simulink model "mvdc_mpc"  (R2018b)
settings: configuration reference "Active" (kept outside this file)
undefined symbols (not defined in the file): A_VehicleReference_m2, acc_control_learning, ax_lim_mps2, ay_lim_mps2, DiscIntNeverNeededParam, drag_coefficient, l_front_m, l_rear_m, LatAcc_cov_debug, LatAcc_FFweights, LatAcc_mean_debug, LongAcc_FFweights, P_VDC_axFFModelLearningEnable, P_VDC_axFFModelLearningRate, P_VDC_axFFModelLearningReg, P_VDC_ayFFModelLearningEnable, P_VDC_ayFFModelLearningRate, P_VDC_ayFFModelLearningReg, P_VDC_Dist_ax_perc, P_VDC_Dist_ay_perc, P_VDC_EnableNumLatErrorDer_b, P_VDC_EnableTubeMPC, P_VDC_EnableUncertaintyLearning, P_VDC_EnableYawRateAccRepl, P_VDC_LatAcc_BetaGain, P_VDC_LatAcc_EnableForesightFF, P_VDC_LatAcc_FF_Ts, P_VDC_LatAcc_Steering_Ts, P_VDC_LatAcc_UndersteerComp_Ts, P_VDC_LatAcc_VehicleDynamics_Ts, P_VDC_LatAccKi, P_VDC_LatAccKi_Lim_perc, P_VDC_LatAccKp_ay, P_VDC_LatAccKp_Delta, P_VDC_LatErrorDer_Ts_s, P_VDC_LongAcc_EnableForesightFF, P_VDC_LongAcc_FB_Ts, P_VDC_LongAcc_FF_Ts, P_VDC_LongAcc_LimFb_N, P_VDC_LongAccKp, P_VDC_MaxTightening, P_VDC_MinVelSlipCalc_mps, P_VDC_PositiveAxLimScale, P_VDC_StabilizerRearSideSlip_rad, P_VDC_SteeringOvalComp_rad, P_VDC_SteeringSteadyStateUndersteerComp_rad, P_VDC_UncertaintyLearningGain, P_VDC_UncertaintyLearningSamples, P_VDC_UncertaintyTarget_perc, P_VDC_VirtualController, Pos, roh_air, sys, tS, tSSlow, TUMHealthStatus, v_mps, vehiclemass_kg
libraries: simulink x31
(part 2 of 2)

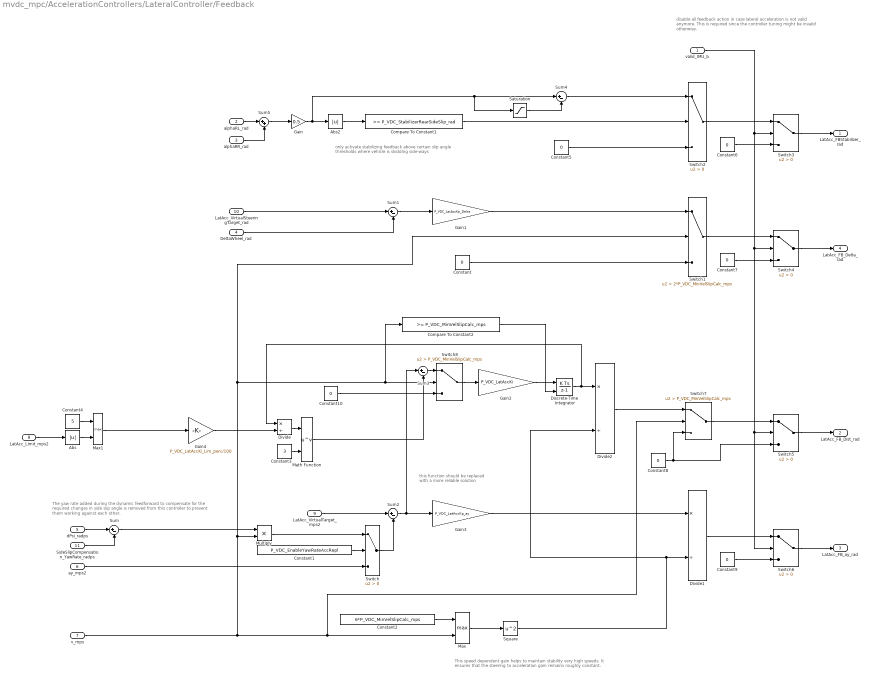
== system mvdc_mpc/AccelerationControllers/LateralController/Feedback ==
  note: disable all feedback action in case
      | lateral acceleration is not valid anymore.
      |
      | This is required since the controller tuning might be invalid otherwise.
  note: only activate stabilizing feedback above certain slip angle
      | thresholds where vehicle is skidding side-ways
  note: this function should be replaced
      | with a more reliable solution
  note: The yaw rate added during the dynamic feedforward to compensate
      | for the required changes in side slip angle is removed from this controller
      | to prevent them working against each other.
  note: This speed dependent gain helps to maintain stability very high speeds.
      | It ensures that the steering to acceleration gain remains roughly constant.
  valid_IMU_b : Inport
  alphaRL_rad : Inport  Port=2
  alphaRR_rad : Inport  Port=3
  DeltaWheel_rad : Inport  Port=4
  dPsi_radps : Inport  Port=5
  ay_mps2 : Inport  Port=6
  v_mps : Inport  Port=7
  LatAcc_Limit_mps2 : Inport  Port=8
  LatAcc_VirtualTarget_mps2 : Inport  Port=9
  LatAcc_VirtualSteeringTarget_rad : Inport  Port=10
  SideSlipCompensation_YawRate_radps : Inport  Port=11
  Abs : Abs
  Abs2 : Abs
  Compare To Constant1 : simulink/Logic and Bit Operations/Compare To Constant  relop=>=  const=P_VDC_StabilizerRearSideSlip_rad  OutDataTypeStr=boolean
  Compare To Constant2 : simulink/Logic and Bit Operations/Compare To Constant  relop=>=  const=P_VDC_MinVelSlipCalc_mps  OutDataTypeStr=boolean
  Constant{,5..10} (7 alike) : Constant  Value=0
  Constant1 : Constant  Value=P_VDC_EnableYawRateAccRepl
  Constant2 : Constant  Value=6*P_VDC_MinVelSlipCalc_mps
  Constant3 : Constant  Value=3
  Constant4 : Constant  Value=5
  Discrete-Time Integrator : DiscreteIntegrator  ExternalReset=falling  SampleTime=-1  ICPrevOutput=DiscIntNeverNeededParam  ICPrevScaledInput=DiscIntNeverNeededParam
  Divide : Product  Inputs=*/
  Divide1 : Product  Inputs=*/
  Divide2 : Product  Inputs=*/
  Gain : Gain  Gain=0.5
  Gain1 : Gain  Gain=P_VDC_LatAccKp_Delta
  Gain2 : Gain  Gain=P_VDC_LatAccKi
  Gain3 : Gain  Gain=P_VDC_LatAccKp_ay
  Gain4 : Gain  Gain=P_VDC_LatAccKi_Lim_perc/100
  Math Function : Math  Operator=pow  SaturateOnIntegerOverflow=on
  Max : MinMax  Function=max  Inputs=2
  Max1 : MinMax  Function=max  Inputs=2
  Multiply : Product
  Saturation : Saturate  UpperLimit=P_VDC_StabilizerRearSideSlip_rad  LowerLimit=-P_VDC_StabilizerRearSideSlip_rad
  Square : Math  Operator=square  SaturateOnIntegerOverflow=on
  Sum{,1..4} (5 alike) : Sum  Inputs=|+-
  Sum5 : Sum  Inputs=|++
  Switch{,2..6} (6 alike) : Switch  Criteria=u2 > Threshold
  Switch1 : Switch  Criteria=u2 > Threshold  Threshold=2*P_VDC_MinVelSlipCalc_mps
  Switch7 : Switch  Criteria=u2 > Threshold  Threshold=P_VDC_MinVelSlipCalc_mps
  Switch8 : Switch  Criteria=u2 > Threshold  Threshold=P_VDC_MinVelSlipCalc_mps
  LatAcc_FBStabilizer_rad : Outport
  LatAcc_FB_Dist_rad : Outport  Port=2
  LatAcc_FB_ay_rad : Outport  Port=3
  LatAcc_FB_Delta_rad : Outport  Port=4
  wires:
  Gain3/1 -> Divide1/1
  Constant2/1 -> Max/1
  Square/1 -> Divide2/2, Divide1/2
  v_mps/1 -> Compare To Constant2/1, Switch8/2, Switch1/2, Multiply/2, Switch7/2, Max/2
  Max/1 -> Square/1
  Multiply/1 -> Switch/1
  ay_mps2/1 -> Switch/3
  Constant1/1 -> Switch/2
  dPsi_radps/1 -> Sum/1
  SideSlipCompensation_YawRate_radps/1 -> Sum/2
  Sum/1 -> Multiply/1
  Switch/1 -> Sum2/2
  LatAcc_VirtualSteeringTarget_rad/1 -> Sum1/1
  DeltaWheel_rad/1 -> Sum1/2
  Sum1/1 -> Gain1/1
  Gain1/1 -> Switch1/1
  Constant/1 -> Switch1/3
  Discrete-Time Integrator/1 -> Divide/1, Divide2/1
  Sum2/1 -> Sum3/1, Gain3/1
  Gain4/1 -> Divide/2
  Divide/1 -> Math Function/1
  Constant3/1 -> Math Function/2
  Max1/1 -> Gain4/1
  Abs/1 -> Max1/2
  LatAcc_VirtualTarget_mps2/1 -> Sum2/1
  Constant4/1 -> Max1/1
  Gain2/1 -> Discrete-Time Integrator/1
  Math Function/1 -> Sum3/2
  Constant5/1 -> Switch2/3
  Abs2/1 -> Compare To Constant1/1
  Sum4/1 -> Switch2/1
  Gain/1 -> Saturation/1, Sum4/1, Abs2/1
  Saturation/1 -> Sum4/2
  Compare To Constant1/1 -> Switch2/2
  LatAcc_Limit_mps2/1 -> Abs/1
  alphaRL_rad/1 -> Sum5/1
  alphaRR_rad/1 -> Sum5/2
  Sum5/1 -> Gain/1
  Switch2/1 -> Switch3/1
  Switch3/1 -> LatAcc_FBStabilizer_rad/1
  Switch1/1 -> Switch4/1
  Switch4/1 -> LatAcc_FB_Delta_rad/1
  Switch5/1 -> LatAcc_FB_Dist_rad/1
  Divide1/1 -> Switch6/1
  Switch6/1 -> LatAcc_FB_ay_rad/1
  valid_IMU_b/1 -> Switch6/2, Switch5/2, Switch4/2, Switch3/2
  Constant6/1 -> Switch3/3
  Constant7/1 -> Switch4/3
  Constant8/1 -> Switch5/3, Switch7/3
  Constant9/1 -> Switch6/3
  Switch7/1 -> Switch5/1
  Divide2/1 -> Switch7/1
  Switch8/1 -> Gain2/1
  Sum3/1 -> Switch8/1
  Constant10/1 -> Switch8/3
  Compare To Constant2/1 -> Discrete-Time Integrator/2

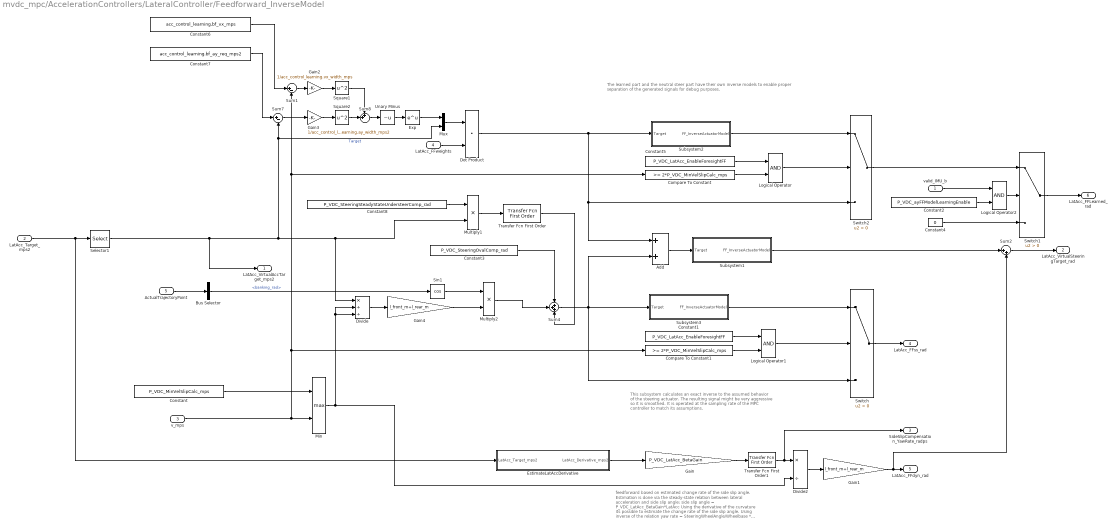
== system mvdc_mpc/AccelerationControllers/LateralController/Feedforward_InverseModel ==
  note: The learned part and the neutral steer part have their own
      | inverse models to enable proper separation of the generated signals for debug purposes.
  note: This subsystem calculates an exact inverse
      | to the assumed behavior of the steering actuator.
      | The resulting signal might be very aggressive so it is smoothed.
      | It is operated at the sampling rate of the MPC controller to match
      | its assumptions.
  note: feedforward based on estimated change rate
      | of the side slip angle. Estimation is done via the steady-state
      | relation between lateral acceleration and side slip angle:
      |
      | side slip angle = P_VDC_LatAcc_BetaGain*LatAcc
      |
      | Using the derivative of the curvature its possible to estimate the
      | change rate of the side slip angle. Using inverse of the relation
      |
      | yaw rate = SteeringWheelAngle/Wheelbase * Velocity
      |
      | we can calculate a compensation yaw rate and the corresponding
      | steering wheel angle.
  valid_IMU_b : Inport
  LatAcc_Target_mps2 : Inport  Port=2
  v_mps : Inport  Port=3
  LatAcc_FFweights : Inport  Port=4
  ActualTrajectoryPoint : Inport  Port=5
  Add : Sum
  Bus Selector : BusSelector  OutputSignals=banking_rad
  Compare To Constant : simulink/Logic and Bit Operations/Compare To Constant  relop=>=  const=2*P_VDC_MinVelSlipCalc_mps  OutDataTypeStr=boolean
  Compare To Constant1 : simulink/Logic and Bit Operations/Compare To Constant  relop=>=  const=2*P_VDC_MinVelSlipCalc_mps  OutDataTypeStr=boolean
  Constant : Constant  Value=P_VDC_MinVelSlipCalc_mps
  Constant1 : Constant  Value=P_VDC_LatAcc_EnableForesightFF
  Constant2 : Constant  Value=P_VDC_ayFFModelLearningEnable
  Constant3 : Constant  Value=P_VDC_SteeringOvalComp_rad
  Constant4 : Constant  Value=0
  Constant5 : Constant  Value=P_VDC_LatAcc_EnableForesightFF
  Constant6 : Constant  Value=acc_control_learning.bf_vx_mps
  Constant7 : Constant  Value=acc_control_learning.bf_ay_req_mps2
  Constant8 : Constant  Value=P_VDC_SteeringSteadyStateUndersteerComp_rad
  Divide : Product  Inputs=*//
  Divide2 : Product  Inputs=*/
  Dot Product : DotProduct  InputSameDT=on  OutDataTypeStr=Inherit: Inherit via internal rule
  EstimateLatAccDerivative : Subsystem
  Exp : Math  SaturateOnIntegerOverflow=on
  Gain : Gain  Gain=P_VDC_LatAcc_BetaGain
  Gain1 : Gain  Gain=l_front_m+l_rear_m
  Gain2 : Gain  Gain=1/acc_control_learning.vx_width_mps
  Gain3 : Gain  Gain=1/acc_control_learning.ay_width_mps2
  Gain4 : Gain  Gain=l_front_m+l_rear_m
  Logical Operator : Logic  AllPortsSameDT=off  OutDataTypeStr=boolean
  Logical Operator1 : Logic  AllPortsSameDT=off  OutDataTypeStr=boolean
  Logical Operator2 : Logic  AllPortsSameDT=off  OutDataTypeStr=boolean
  Min : MinMax  Function=max  Inputs=2
  Multiply1 : Product
  Multiply2 : Product
  Mux : Mux  Inputs=2
  Selector1 : Selector  InputPortWidth=sys.N_hor+1  IndexOptions=Index vector (dialog)  Indices=1  OutputSizes=1
  Sin1 : Trigonometry  Operator=cos
  Square1 : Math  Operator=square  SaturateOnIntegerOverflow=on
  Square2 : Math  Operator=square  SaturateOnIntegerOverflow=on
  Subsystem1 : Subsystem  SystemSampleTime=tSSlow
  Subsystem2 : Subsystem  SystemSampleTime=tSSlow
  Subsystem3 : Subsystem  SystemSampleTime=tSSlow
  Sum1 : Sum  Inputs=|+-
  Sum2 : Sum  Inputs=|++
  Sum4 : Sum  Inputs=+++
  Sum7 : Sum  Inputs=|+-
  Sum8 : Sum  Inputs=++|
  Switch : Switch  Criteria=u2 > Threshold
  Switch1 : Switch  Criteria=u2 > Threshold
  Switch2 : Switch  Criteria=u2 > Threshold
  Transfer Fcn First Order : simulink/Discrete/Transfer Fcn First Order  PoleZ=exp(-tS/P_VDC_LatAcc_UndersteerComp_Ts)  ICPrevOutput=0.0  DoSatur=off
      settings: SourceProductName=Simulink
  Transfer Fcn First Order1 : simulink/Discrete/Transfer Fcn First Order  PoleZ=exp(-tS/P_VDC_LatAcc_FF_Ts)  ICPrevOutput=0.0  DoSatur=off
      settings: SourceProductName=Simulink
  Unary Minus : UnaryMinus
  LatAcc_VirtualAccTarget_mps2 : Outport
  LatAcc_VirtualSteeringTarget_rad : Outport  Port=2
  SideSlipCompensation_YawRate_radps : Outport  Port=3
  LatAcc_FFss_rad : Outport  Port=4
  LatAcc_FFdyn_rad : Outport  Port=5
  LatAcc_FFLearned_rad : Outport  Port=6
  wires:
  Constant/1 -> Min/1
  LatAcc_Target_mps2/1 -> Selector1/1, EstimateLatAccDerivative/1(LatAcc_Target_mps2)
  Logical Operator1/1 -> Switch/2
  EstimateLatAccDerivative/1(LatAcc_Derivative_mps2) -> Gain/1
  Min/1 -> Divide2/2, Divide/3, Divide/2
  Transfer Fcn First Order1/1 -> SideSlipCompensation_YawRate_radps/1, Divide2/1
  Divide/1 -> Gain4/1
  Divide2/1 -> Gain1/1
  Gain/1 -> Transfer Fcn First Order1/1
  Gain1/1 -> Sum2/2, LatAcc_FFdyn_rad/1
  Switch1/1 -> LatAcc_FFLearned_rad/1
  Constant4/1 -> Switch1/3
  Switch/1 -> LatAcc_FFss_rad/1
  Subsystem2/1(FF_InverseActuatorModel) -> Switch2/1
  Dot Product/1 -> Subsystem2/1(Target), Add/1, Switch2/3
  Switch2/1 -> Switch1/1
  Square1/1 -> Sum8/1
  Sum8/1 -> Unary Minus/1
  Gain3/1 -> Square2/1
  Gain2/1 -> Square1/1
  Square2/1 -> Sum8/2
  LatAcc_FFweights/1 -> Dot Product/2
  Sum1/1 -> Gain2/1
  Sum7/1 -> Gain3/1
  Unary Minus/1 -> Exp/1
  Exp/1 -> Mux/1
  Constant6/1 -> Sum1/1
  Constant7/1 -> Sum7/1
  v_mps/1 -> Min/2, Compare To Constant1/1, Compare To Constant/1, Sum1/2
  Mux/1 -> Dot Product/1
  Sum4/1 -> Subsystem3/1(Target), Add/2, Switch/3
  Subsystem3/1(FF_InverseActuatorModel) -> Switch/1
  Subsystem1/1(FF_InverseActuatorModel) -> Sum2/1
  Add/1 -> Subsystem1/1(Target)
  Sum2/1 -> LatAcc_VirtualSteeringTarget_rad/1
  Constant5/1 -> Logical Operator/1
  Logical Operator/1 -> Switch2/2
  Compare To Constant/1 -> Logical Operator/2
  Constant1/1 -> Logical Operator1/1
  Compare To Constant1/1 -> Logical Operator1/2
  Logical Operator2/1 -> Switch1/2
  Constant2/1 -> Logical Operator2/2
  valid_IMU_b/1 -> Logical Operator2/1
  Constant3/1 -> Sum4/1
  Constant8/1 -> Multiply1/1
  Multiply1/1 -> Transfer Fcn First Order/1
  Transfer Fcn First Order/1 -> Sum4/3
  ActualTrajectoryPoint/1 -> Bus Selector/1
  Selector1/1 -> LatAcc_VirtualAccTarget_mps2/1, Sum7/2, Mux/2, Multiply1/2, Divide/1  "Target"
  Gain4/1 -> Multiply2/2
  Multiply2/1 -> Sum4/2
  Sin1/1 -> Multiply2/1
  Bus Selector/1 -> Sin1/1  "<banking_rad>"

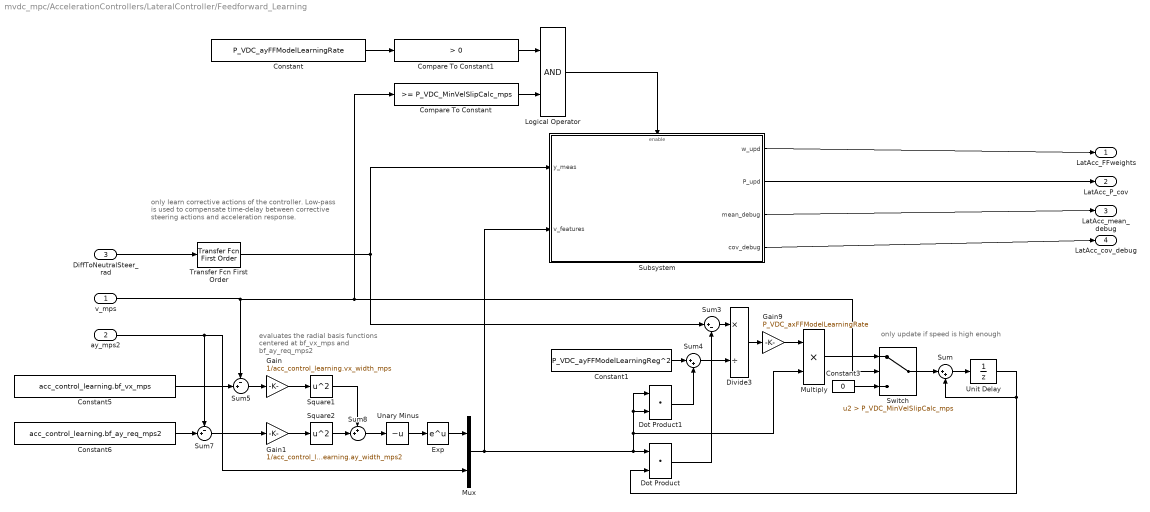
== system mvdc_mpc/AccelerationControllers/LateralController/Feedforward_Learning ==
  note: evaluates the radial
      | basis functions centered at
      | bf_vx_mps and bf_ay_req_mps2
  note: only learn corrective actions of the controller.
      | Low-pass is used to compensate time-delay
      | between corrective steering actions and acceleration
      | response.
  note: only update if speed is high enough
  v_mps : Inport
  ay_mps2 : Inport  Port=2
  DiffToNeutralSteer_rad : Inport  Port=3
  Compare To Constant : simulink/Logic and Bit Operations/Compare To Constant  relop=>=  const=P_VDC_MinVelSlipCalc_mps  OutDataTypeStr=boolean
  Compare To Constant1 : simulink/Logic and Bit Operations/Compare To Constant  relop=>  const=0  OutDataTypeStr=boolean
  Constant : Constant  Value=P_VDC_ayFFModelLearningRate
  Constant1 : Constant  Value=P_VDC_ayFFModelLearningReg^2
  Constant3 : Constant  Value=0
  Constant5 : Constant  Value=acc_control_learning.bf_vx_mps
  Constant6 : Constant  Value=acc_control_learning.bf_ay_req_mps2
  Divide3 : Product  Inputs=*/
  Dot Product : DotProduct  InputSameDT=on  OutDataTypeStr=Inherit: Inherit via internal rule
  Dot Product1 : DotProduct  InputSameDT=on  OutDataTypeStr=Inherit: Inherit via internal rule
  Exp : Math  SaturateOnIntegerOverflow=on
  Gain : Gain  Gain=1/acc_control_learning.vx_width_mps
  Gain1 : Gain  Gain=1/acc_control_learning.ay_width_mps2
  Gain9 : Gain  Gain=P_VDC_axFFModelLearningRate
  Logical Operator : Logic  AllPortsSameDT=off  OutDataTypeStr=boolean
  Multiply : Product
  Mux : Mux  Inputs=2
  Square1 : Math  Operator=square  SaturateOnIntegerOverflow=on
  Square2 : Math  Operator=square  SaturateOnIntegerOverflow=on
  Subsystem : Subsystem
  Sum : Sum  Inputs=|++
  Sum3 : Sum  Inputs=|+-
  Sum4 : Sum  Inputs=|++
  Sum5 : Sum  Inputs=-+|
  Sum7 : Sum  Inputs=-+|
  Sum8 : Sum  Inputs=++|
  Switch : Switch  Criteria=u2 > Threshold  Threshold=P_VDC_MinVelSlipCalc_mps
  Transfer Fcn First Order : simulink/Discrete/Transfer Fcn First Order  PoleZ=exp(-tS/P_VDC_LatAcc_Steering_Ts)  ICPrevOutput=0.0  DoSatur=off
      settings: SourceProductName=Simulink
  Unary Minus : UnaryMinus
  Unit Delay : UnitDelay  InitialCondition=acc_control_learning.w0  SampleTime=-1
  LatAcc_FFweights : Outport
  LatAcc_P_cov : Outport  Port=2
  LatAcc_mean_debug : Outport  Port=3
  LatAcc_cov_debug : Outport  Port=4
  wires:
  Unary Minus/1 -> Exp/1
  Mux/1 -> Subsystem/2(v_features), Dot Product1/1, Dot Product1/2, Multiply/2, Dot Product/1
  Switch/1 -> Sum/1
  Sum/1 -> Unit Delay/1
  v_mps/1 -> Sum5/1, Compare To Constant/1, Switch/2
  Square2/1 -> Sum8/2
  Sum4/1 -> Divide3/2
  Constant1/1 -> Sum4/1
  Dot Product1/1 -> Sum4/2
  Constant5/1 -> Sum5/2
  Multiply/1 -> Switch/1
  Dot Product/1 -> Sum3/2
  Sum5/1 -> Gain/1
  Gain/1 -> Square1/1
  Unit Delay/1 -> Sum/2, Dot Product/2
  Divide3/1 -> Gain9/1
  Sum8/1 -> Unary Minus/1
  Sum7/1 -> Gain1/1
  ay_mps2/1 -> Mux/2, Sum7/1
  DiffToNeutralSteer_rad/1 -> Transfer Fcn First Order/1
  Gain9/1 -> Multiply/1
  Constant3/1 -> Switch/3
  Square1/1 -> Sum8/1
  Constant6/1 -> Sum7/2
  Gain1/1 -> Square2/1
  Sum3/1 -> Divide3/1
  Transfer Fcn First Order/1 -> Subsystem/1(y_meas), Sum3/1
  Exp/1 -> Mux/1
  Subsystem/1(w_upd) -> LatAcc_FFweights/1
  Subsystem/2(P_upd) -> LatAcc_P_cov/1
  Subsystem/3(mean_debug) -> LatAcc_mean_debug/1
  Subsystem/4(cov_debug) -> LatAcc_cov_debug/1
  Constant/1 -> Compare To Constant1/1
  Compare To Constant/1 -> Logical Operator/2
  Compare To Constant1/1 -> Logical Operator/1
  Logical Operator/1 -> Subsystem/Enable

== system mvdc_mpc/AccelerationControllers/LongitudinalController/Feedforward_Aero ==
  v_mps : Inport
  Gain2 : Gain  Gain=drag_coefficient
  Gain3 : Gain  Gain=roh_air
  Gain4 : Gain  Gain=0.5
  Gain7 : Gain  Gain=A_VehicleReference_m2
  Product : Product
  LongAcc_FFdist_N : Outport
  wires:
  Gain2/1 -> Gain7/1
  v_mps/1 -> Product/2, Product/1
  Product/1 -> Gain2/1
  Gain3/1 -> Gain4/1
  Gain7/1 -> Gain3/1
  Gain4/1 -> LongAcc_FFdist_N/1

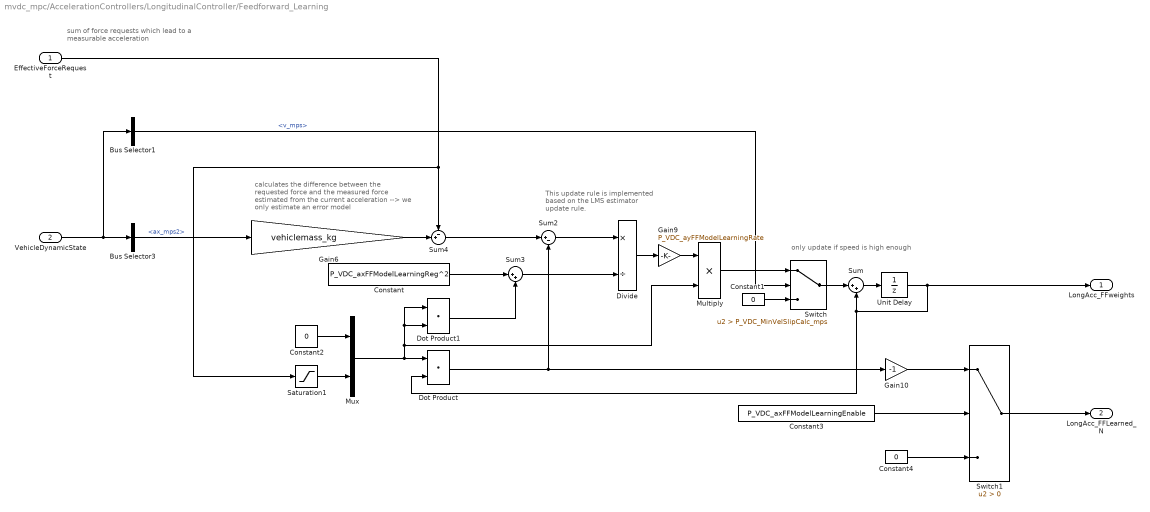
== system mvdc_mpc/AccelerationControllers/LongitudinalController/Feedforward_Learning ==
  note: only update if speed is high enough
  note: sum of force requests
      | which lead to a measurable acceleration
  note: This update rule is implemented based on the LMS estimator
      | update rule.
  note: calculates the difference between
      | the requested force and the measured force
      | estimated from the current acceleration
      | --> we only estimate an error model
  EffectiveForceRequest : Inport
  VehicleDynamicState : Inport  Port=2
  Bus Selector1 : BusSelector  OutputSignals=v_mps
  Bus Selector3 : BusSelector  OutputSignals=ax_mps2
  Constant : Constant  Value=P_VDC_axFFModelLearningReg^2
  Constant1 : Constant  Value=0
  Constant2 : Constant  Value=0
  Constant3 : Constant  Value=P_VDC_axFFModelLearningEnable
  Constant4 : Constant  Value=0
  Divide : Product  Inputs=*/
  Dot Product : DotProduct  InputSameDT=on  OutDataTypeStr=Inherit: Inherit via internal rule
  Dot Product1 : DotProduct  InputSameDT=on  OutDataTypeStr=Inherit: Inherit via internal rule
  Gain10 : Gain  Gain=-1
  Gain6 : Gain  Gain=vehiclemass_kg
  Gain9 : Gain  Gain=P_VDC_ayFFModelLearningRate
  Multiply : Product
  Mux : Mux  Inputs=2
  Saturation1 : Saturate  UpperLimit=0  LowerLimit=-inf
  Sum : Sum  Inputs=|++
  Sum2 : Sum  Inputs=|+-
  Sum3 : Sum  Inputs=|++
  Sum4 : Sum  Inputs=-+|
  Switch : Switch  Criteria=u2 > Threshold  Threshold=P_VDC_MinVelSlipCalc_mps
  Switch1 : Switch  Criteria=u2 > Threshold
  Unit Delay : UnitDelay  InitialCondition=[0; 0]  SampleTime=-1
  LongAcc_FFweights : Outport
  LongAcc_FFLearned_N : Outport  Port=2
  wires:
  Switch/1 -> Sum/1
  EffectiveForceRequest/1 -> Saturation1/1, Sum4/1
  Constant/1 -> Sum3/1
  Gain9/1 -> Multiply/1
  Bus Selector3/1 -> Gain6/1  "<ax_mps2>"
  Unit Delay/1 -> LongAcc_FFweights/1, Sum/2, Dot Product/2
  Divide/1 -> Gain9/1
  Constant2/1 -> Mux/1
  Gain6/1 -> Sum4/2
  Multiply/1 -> Switch/1
  Constant1/1 -> Switch/3
  Dot Product1/1 -> Sum3/2
  Sum2/1 -> Divide/1
  Sum4/1 -> Sum2/1
  Dot Product/1 -> Gain10/1, Sum2/2
  Sum3/1 -> Divide/2
  Mux/1 -> Multiply/2, Dot Product1/1, Dot Product1/2, Dot Product/1
  Sum/1 -> Unit Delay/1
  Saturation1/1 -> Mux/2
  VehicleDynamicState/1 -> Bus Selector1/1, Bus Selector3/1
  Bus Selector1/1 -> Switch/2  "<v_mps>"
  Gain10/1 -> Switch1/1
  Switch1/1 -> LongAcc_FFLearned_N/1
  Constant3/1 -> Switch1/2
  Constant4/1 -> Switch1/3

== system mvdc_mpc/AccelerationControllers/LongitudinalController/Feedforward_LongAcc ==
  note: The upper path uses an exponentially weighted look-ahead
      | of the acceleration calculated by the TMPC to generate
      | appropriate feedforward commands and deal with actuator delay
      | and neglected vehicle dynamics.
      |
      | The lower path uses only the current value.
  LongAcc_Target_mps2 : Inport
  Constant1 : Constant  Value=P_VDC_LongAcc_EnableForesightFF
  Gain : Gain  Gain=exp(-tSSlow/P_VDC_LongAcc_FF_Ts*(0:1:sys.N_hor))/sum(exp(-tSSlow/P_VDC_LongAcc_FF_Ts*(0:1:sys.N_hor)))  Multiplication=Matrix(K*u) (u vector)
  Gain1 : Gain  Gain=vehiclemass_kg
  Selector1 : Selector  InputPortWidth=sys.N_hor+1  IndexOptions=Index vector (dialog)  Indices=1  OutputSizes=1
  Switch : Switch  Criteria=u2 > Threshold
  LongAcc_TargetFF_mps2 : Outport
  LongAcc_FFax_N : Outport  Port=2
  wires:
  Gain1/1 -> LongAcc_FFax_N/1
  LongAcc_Target_mps2/1 -> Selector1/1, Gain/1
  Constant1/1 -> Switch/2
  Selector1/1 -> Switch/3
  Switch/1 -> LongAcc_TargetFF_mps2/1, Gain1/1
  Gain/1 -> Switch/1

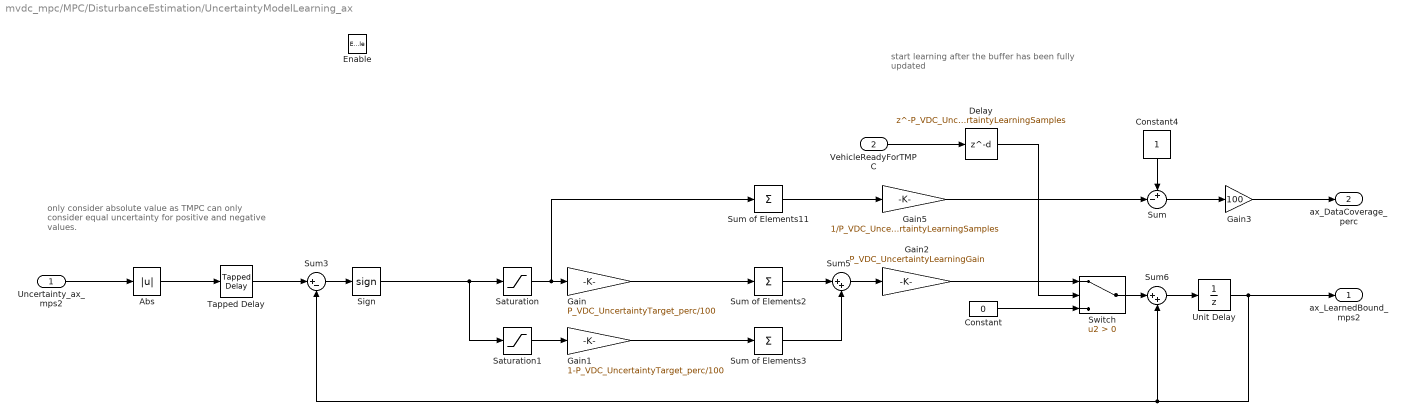
== system mvdc_mpc/MPC/DisturbanceEstimation/UncertaintyModelLearning_ax ==
  note: only consider absolute
      | value as TMPC can only consider
      | equal uncertainty for positive and negative values.
  note: start learning after the buffer has been fully updated
  Uncertainty_ax_mps2 : Inport
  VehicleReadyForTMPC : Inport  Port=2
  Enable : EnablePort
  Abs : Abs
  Constant : Constant  Value=0
  Constant4 : Constant
  Delay : Delay  DelayLength=P_VDC_UncertaintyLearningSamples
  Gain : Gain  Gain=P_VDC_UncertaintyTarget_perc/100
  Gain1 : Gain  Gain=1-P_VDC_UncertaintyTarget_perc/100
  Gain2 : Gain  Gain=P_VDC_UncertaintyLearningGain
  Gain3 : Gain  Gain=100
  Gain5 : Gain  Gain=1/P_VDC_UncertaintyLearningSamples
  Saturation : Saturate  UpperLimit=inf  LowerLimit=0
  Saturation1 : Saturate  UpperLimit=0  LowerLimit=-inf
  Sign : Signum
  Sum : Sum  Inputs=+-|
  Sum of Elements11 : Sum  Inputs=+
  Sum of Elements2 : Sum  Inputs=+
  Sum of Elements3 : Sum  Inputs=+
  Sum3 : Sum  Inputs=|+-
  Sum5 : Sum  Inputs=|++
  Sum6 : Sum  Inputs=|++
  Switch : Switch  Criteria=u2 > Threshold
  Tapped Delay : simulink/Discrete/Tapped Delay  vinit=0  samptime=-1  NumDelays=P_VDC_UncertaintyLearningSamples  DelayOrder=Oldest  includeCurrent=on
  Unit Delay : UnitDelay  SampleTime=-1
  ax_LearnedBound_mps2 : Outport
  ax_DataCoverage_perc : Outport  Port=2
  wires:
  Sign/1 -> Saturation1/1, Saturation/1
  Gain/1 -> Sum of Elements2/1
  Saturation/1 -> Gain/1, Sum of Elements11/1
  Sum of Elements2/1 -> Sum5/1
  Sum3/1 -> Sign/1
  Gain1/1 -> Sum of Elements3/1
  Saturation1/1 -> Gain1/1
  Sum of Elements3/1 -> Sum5/2
  Uncertainty_ax_mps2/1 -> Abs/1
  Tapped Delay/1 -> Sum3/1
  Constant4/1 -> Sum/1
  Gain5/1 -> Sum/2
  Sum of Elements11/1 -> Gain5/1
  Sum/1 -> Gain3/1
  Gain3/1 -> ax_DataCoverage_perc/1
  VehicleReadyForTMPC/1 -> Delay/1
  Unit Delay/1 -> ax_LearnedBound_mps2/1, Sum6/2, Sum3/2
  Sum5/1 -> Gain2/1
  Sum6/1 -> Unit Delay/1
  Switch/1 -> Sum6/1
  Gain2/1 -> Switch/1
  Constant/1 -> Switch/3
  Delay/1 -> Switch/2
  Abs/1 -> Tapped Delay/1

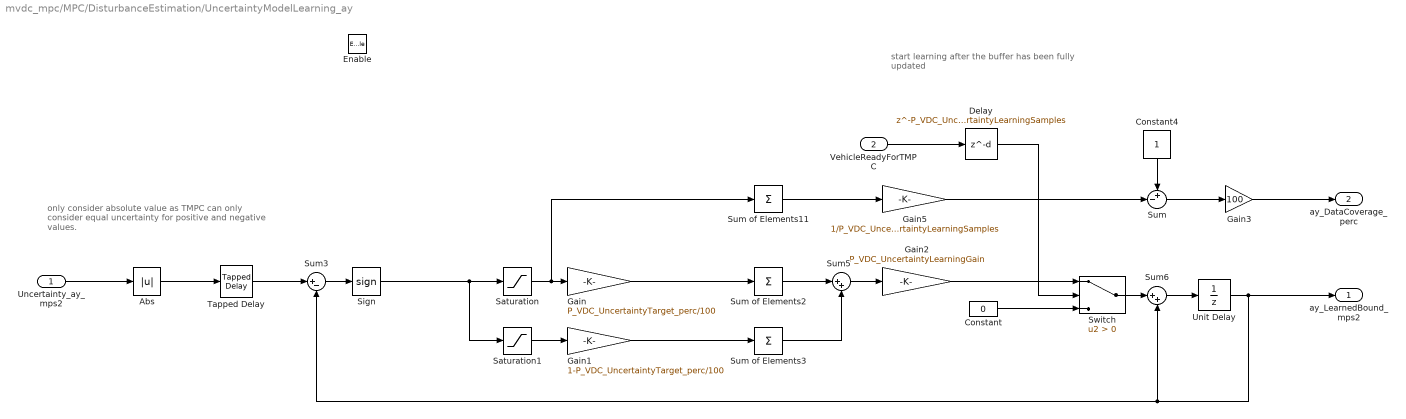
== system mvdc_mpc/MPC/DisturbanceEstimation/UncertaintyModelLearning_ay ==
  note: only consider absolute
      | value as TMPC can only consider
      | equal uncertainty for positive and negative values.
  note: start learning after the buffer has been fully updated
  Uncertainty_ay_mps2 : Inport
  VehicleReadyForTMPC : Inport  Port=2
  Enable : EnablePort
  Abs : Abs
  Constant : Constant  Value=0
  Constant4 : Constant
  Delay : Delay  DelayLength=P_VDC_UncertaintyLearningSamples
  Gain : Gain  Gain=P_VDC_UncertaintyTarget_perc/100
  Gain1 : Gain  Gain=1-P_VDC_UncertaintyTarget_perc/100
  Gain2 : Gain  Gain=P_VDC_UncertaintyLearningGain
  Gain3 : Gain  Gain=100
  Gain5 : Gain  Gain=1/P_VDC_UncertaintyLearningSamples
  Saturation : Saturate  UpperLimit=inf  LowerLimit=0
  Saturation1 : Saturate  UpperLimit=0  LowerLimit=-inf
  Sign : Signum
  Sum : Sum  Inputs=+-|
  Sum of Elements11 : Sum  Inputs=+
  Sum of Elements2 : Sum  Inputs=+
  Sum of Elements3 : Sum  Inputs=+
  Sum3 : Sum  Inputs=|+-
  Sum5 : Sum  Inputs=|++
  Sum6 : Sum  Inputs=|++
  Switch : Switch  Criteria=u2 > Threshold
  Tapped Delay : simulink/Discrete/Tapped Delay  vinit=0  samptime=-1  NumDelays=P_VDC_UncertaintyLearningSamples  DelayOrder=Oldest  includeCurrent=on
  Unit Delay : UnitDelay  SampleTime=-1
  ay_LearnedBound_mps2 : Outport
  ay_DataCoverage_perc : Outport  Port=2
  wires:
  Sign/1 -> Saturation1/1, Saturation/1
  Gain/1 -> Sum of Elements2/1
  Saturation/1 -> Gain/1, Sum of Elements11/1
  Sum of Elements2/1 -> Sum5/1
  Sum3/1 -> Sign/1
  Gain1/1 -> Sum of Elements3/1
  Saturation1/1 -> Gain1/1
  Sum of Elements3/1 -> Sum5/2
  Uncertainty_ay_mps2/1 -> Abs/1
  Tapped Delay/1 -> Sum3/1
  Constant4/1 -> Sum/1
  Gain5/1 -> Sum/2
  Sum of Elements11/1 -> Gain5/1
  Sum/1 -> Gain3/1
  Gain3/1 -> ay_DataCoverage_perc/1
  VehicleReadyForTMPC/1 -> Delay/1
  Unit Delay/1 -> ay_LearnedBound_mps2/1, Sum6/2, Sum3/2
  Sum5/1 -> Gain2/1
  Sum6/1 -> Unit Delay/1
  Switch/1 -> Sum6/1
  Gain2/1 -> Switch/1
  Constant/1 -> Switch/3
  Delay/1 -> Switch/2
  Abs/1 -> Tapped Delay/1

== system mvdc_mpc/MPC/TubeMPC/Subsystem ==
  note: parse solver status
      | 1 --> osqp_solved --> alright
      | 2 --> osqp_max_iter_reached --> we use iterations to limit execution time, therefore also alright
      | -1 --> osqp_solved_inaccurate --> also alright to tolerate not so good solutions
  status : Inport
  Compare To Constant : simulink/Logic and Bit Operations/Compare To Constant  relop===  const=1  OutDataTypeStr=boolean
  Compare To Constant1 : simulink/Logic and Bit Operations/Compare To Constant  relop===  const=2  OutDataTypeStr=boolean
  Compare To Constant2 : simulink/Logic and Bit Operations/Compare To Constant  relop===  const=-2  OutDataTypeStr=boolean
  Logical Operator : Logic  Operator=OR  Inputs=3  AllPortsSameDT=off  OutDataTypeStr=boolean
  solver_ok : Outport
  wires:
  status/1 -> Compare To Constant2/1, Compare To Constant1/1, Compare To Constant/1
  Compare To Constant1/1 -> Logical Operator/2
  Compare To Constant/1 -> Logical Operator/1
  Compare To Constant2/1 -> Logical Operator/3
  Logical Operator/1 -> solver_ok/1

== system mvdc_mpc/MPC/TubeMPC/Subsystem1 ==
  VehicleDynamicState : Inport
  PathPos : Inport  Port=2
  Bus Selector : BusSelector  OutputSignals=psi_rad
  Bus Selector1 : BusSelector  OutputSignals=beta_rad,v_mps
  Bus Selector2 : BusSelector  OutputSignals=d_m
  Discrete Derivative : simulink/Discrete/Discrete Derivative  gainval=1.0  ICPrevScaledInput=0.0  OutMin=[]  OutMax=[]  OutDataType=fixdt(1, 16)  OutScaling=2^-10  DoSatur=off
  Multiply : Product
  Sin : Trigonometry
  Sum : Sum  Inputs=|++
  Transfer Fcn First Order : simulink/Discrete/Transfer Fcn First Order  PoleZ=exp(-tS/P_VDC_LatErrorDer_Ts_s)  ICPrevOutput=0.0  DoSatur=off
      settings: SourceProductName=Simulink
  dot_d_analytical_mps : Outport
  dot_d_numerical_mps : Outport  Port=2
  wires:
  PathPos/1 -> Bus Selector2/1, Bus Selector/1
  VehicleDynamicState/1 -> Bus Selector1/1
  Bus Selector/1 -> Sum/1  "<psi_rad>"
  Bus Selector1/1 -> Sum/2  "<beta_rad>"
  Sum/1 -> Sin/1
  Sin/1 -> Multiply/1
  Bus Selector1/2 -> Multiply/2  "<v_mps>"
  Multiply/1 -> dot_d_analytical_mps/1
  Bus Selector2/1 -> Discrete Derivative/1  "<d_m>"
  Transfer Fcn First Order/1 -> dot_d_numerical_mps/1
  Discrete Derivative/1 -> Transfer Fcn First Order/1

== system mvdc_mpc/AccelerationControllers/LateralController/Feedforward_InverseModel/EstimateLatAccDerivative ==
  LatAcc_Target_mps2 : Inport
  Gain2 : Gain  Gain=1/tSSlow
  Selector2 : Selector  InputPortWidth=sys.N_hor+1  IndexOptions=Index vector (dialog)  Indices=2  OutputSizes=1
  Selector3 : Selector  InputPortWidth=sys.N_hor+1  IndexOptions=Index vector (dialog)  Indices=1  OutputSizes=1
  Sum1 : Sum  Inputs=|+-
  LatAcc_Derivative_mps2 : Outport
  wires:
  Gain2/1 -> LatAcc_Derivative_mps2/1
  LatAcc_Target_mps2/1 -> Selector3/1, Selector2/1
  Selector2/1 -> Sum1/1
  Selector3/1 -> Sum1/2
  Sum1/1 -> Gain2/1

== system mvdc_mpc/AccelerationControllers/LateralController/Feedforward_InverseModel/Subsystem1 ==
  note: Model Inversion
  note: Steering Actuator Forward Simulation
  Target : Inport
  Gain1 : Gain  Gain=exp(-tS/(P_VDC_LatAcc_Steering_Ts+P_VDC_LatAcc_VehicleDynamics_Ts))
  Gain2 : Gain  Gain=1-exp(-tS/(P_VDC_LatAcc_Steering_Ts+P_VDC_LatAcc_VehicleDynamics_Ts))
  Gain3 : Gain  Gain=1/(1-exp(-tS/(P_VDC_LatAcc_Steering_Ts+P_VDC_LatAcc_VehicleDynamics_Ts)))
  Sum : Sum  Inputs=|++
  Sum1 : Sum  Inputs=|+-
  Transfer Fcn First Order1 : simulink/Discrete/Transfer Fcn First Order  PoleZ=exp(-tS/P_VDC_LatAcc_FF_Ts)  ICPrevOutput=0.0  DoSatur=off
      settings: SourceProductName=Simulink
  Unit Delay : UnitDelay  SampleTime=-1
  FF_InverseActuatorModel : Outport
  wires:
  Unit Delay/1 -> Gain1/1
  Gain2/1 -> Sum/1
  Gain3/1 -> Transfer Fcn First Order1/1, Gain2/1
  Sum1/1 -> Gain3/1
  Target/1 -> Sum1/1
  Gain1/1 -> Sum1/2, Sum/2
  Sum/1 -> Unit Delay/1
  Transfer Fcn First Order1/1 -> FF_InverseActuatorModel/1

== system mvdc_mpc/AccelerationControllers/LateralController/Feedforward_InverseModel/Subsystem2 ==
  note: Model Inversion
  note: Steering Actuator Forward Simulation
  Target : Inport
  Gain1 : Gain  Gain=exp(-tS/(P_VDC_LatAcc_Steering_Ts+P_VDC_LatAcc_VehicleDynamics_Ts))
  Gain2 : Gain  Gain=1-exp(-tS/(P_VDC_LatAcc_Steering_Ts+P_VDC_LatAcc_VehicleDynamics_Ts))
  Gain3 : Gain  Gain=1/(1-exp(-tS/(P_VDC_LatAcc_Steering_Ts+P_VDC_LatAcc_VehicleDynamics_Ts)))
  Sum : Sum  Inputs=|++
  Sum1 : Sum  Inputs=|+-
  Transfer Fcn First Order1 : simulink/Discrete/Transfer Fcn First Order  PoleZ=exp(-tS/P_VDC_LatAcc_FF_Ts)  ICPrevOutput=0.0  DoSatur=off
      settings: SourceProductName=Simulink
  Unit Delay : UnitDelay  SampleTime=-1
  FF_InverseActuatorModel : Outport
  wires:
  Unit Delay/1 -> Gain1/1
  Gain2/1 -> Sum/1
  Gain3/1 -> Transfer Fcn First Order1/1, Gain2/1
  Sum1/1 -> Gain3/1
  Target/1 -> Sum1/1
  Gain1/1 -> Sum1/2, Sum/2
  Sum/1 -> Unit Delay/1
  Transfer Fcn First Order1/1 -> FF_InverseActuatorModel/1

== system mvdc_mpc/AccelerationControllers/LateralController/Feedforward_InverseModel/Subsystem3 ==
  note: Model Inversion
  note: Steering Actuator Forward Simulation
  Target : Inport
  Gain1 : Gain  Gain=exp(-tS/(P_VDC_LatAcc_Steering_Ts+P_VDC_LatAcc_VehicleDynamics_Ts))
  Gain2 : Gain  Gain=1-exp(-tS/(P_VDC_LatAcc_Steering_Ts+P_VDC_LatAcc_VehicleDynamics_Ts))
  Gain3 : Gain  Gain=1/(1-exp(-tS/(P_VDC_LatAcc_Steering_Ts+P_VDC_LatAcc_VehicleDynamics_Ts)))
  Sum : Sum  Inputs=|++
  Sum1 : Sum  Inputs=|+-
  Transfer Fcn First Order1 : simulink/Discrete/Transfer Fcn First Order  PoleZ=exp(-tS/P_VDC_LatAcc_FF_Ts)  ICPrevOutput=0.0  DoSatur=off
      settings: SourceProductName=Simulink
  Unit Delay : UnitDelay  SampleTime=-1
  FF_InverseActuatorModel : Outport
  wires:
  Unit Delay/1 -> Gain1/1
  Gain2/1 -> Sum/1
  Gain3/1 -> Transfer Fcn First Order1/1, Gain2/1
  Sum1/1 -> Gain3/1
  Target/1 -> Sum1/1
  Gain1/1 -> Sum1/2, Sum/2
  Sum/1 -> Unit Delay/1
  Transfer Fcn First Order1/1 -> FF_InverseActuatorModel/1

== system mvdc_mpc/AccelerationControllers/LateralController/Feedforward_Learning/Subsystem ==
  y_meas : Inport
  v_features : Inport  Port=2
  Enable : EnablePort
  MATLAB Function : MATLAB Function  TreatAsAtomicUnit=on
  Unit Delay1 : UnitDelay  InitialCondition=1e-10*eye(length(acc_control_learning.w0))  SampleTime=-1
  Unit Delay2 : UnitDelay  InitialCondition=acc_control_learning.w0  SampleTime=-1
  w_upd : Outport  InitialOutput=acc_control_learning.w0
  P_upd : Outport  Port=2  InitialOutput=1e-10*eye(length(acc_control_learning.w0))
  mean_debug : Outport  Port=3
  cov_debug : Outport  Port=4
  wires:
  MATLAB Function/2(P_upd) -> Unit Delay1/1, P_upd/1
  MATLAB Function/1(w_upd) -> Unit Delay2/1, w_upd/1
  Unit Delay1/1 -> MATLAB Function/4(P_old)
  Unit Delay2/1 -> MATLAB Function/3(w_old)
  v_features/1 -> MATLAB Function/1(v)
  y_meas/1 -> MATLAB Function/2(y_meas)
  MATLAB Function/3(mean_debug) -> mean_debug/1
  MATLAB Function/4(cov_debug) -> cov_debug/1

== matlab function mvdc_mpc/MPC/TubeMPC/transformMPCResult ==
  data: status input; u_opt_total output; x_pred_m output size=sys.N_hor+1; y_pred_m output size=sys.N_hor+1; u_opt_total input; errorState input; x_traj input; y_traj input; psi_traj input; v_traj input; ax_diff_traj input; d_Target_m input; ax_lim_mps2 input; ay_lim_mps2 input; vx_lin_mps input; kappa_lin_radpm input; UncertaintyTube input; vx_pred_mps output size=sys.N_hor+1; x_pred_left_m output; y_pred_left_m output; x_pred_right_m output; y_pred_right_m output; d_pred_m output size=sys.N_hor+1; dot_d_pred_mps output size=sys.N_hor+1; s_dot_pred_mps output size=sys.N_hor+1; ax_pred_mps2 output; ax_tire_pred_mps2 output; ay_pred_mps2 output; TireUtilizationTarget output; cost_values output; sys parameter; drag_coefficient parameter; roh_air parameter; vehiclemass_kg parameter; P_VDC_PositiveAxLimScale parameter
function [u_opt_total, x_pred_m, y_pred_m, vx_pred_mps, ...
    x_pred_left_m, y_pred_left_m, x_pred_right_m, y_pred_right_m,...
    d_pred_m, dot_d_pred_mps, s_dot_pred_mps, ...
    ax_pred_mps2, ax_tire_pred_mps2, ay_pred_mps2, TireUtilizationTarget, cost_values]  = ...
    transformMPCResult(status, u_opt_total, errorState, x_traj, y_traj, ...
    psi_traj, v_traj, ax_diff_traj, d_Target_m, ax_lim_mps2, ay_lim_mps2, ...
    vx_lin_mps, kappa_lin_radpm, UncertaintyTube, ... 
    sys, drag_coefficient, roh_air, vehiclemass_kg, P_VDC_PositiveAxLimScale) ...

[u_opt_total, x_pred_m, y_pred_m, x_pred_left_m, y_pred_left_m, x_pred_right_m, y_pred_right_m, ...
    vx_pred_mps, d_pred_m, dot_d_pred_mps, s_dot_pred_mps, ...
    ax_pred_mps2, ax_tire_pred_mps2, ay_pred_mps2, TireUtilizationTarget, cost_values]  = ...
    transformMPCResult(status, u_opt_total, errorState, x_traj, y_traj, ...
    psi_traj, v_traj, ax_diff_traj, d_Target_m,  ax_lim_mps2, ay_lim_mps2, ...
    vx_lin_mps, kappa_lin_radpm, UncertaintyTube, ...
    sys, drag_coefficient, roh_air, vehiclemass_kg, P_VDC_PositiveAxLimScale);

== matlab function mvdc_mpc/MPC/TubeMPC/prepareOptimizationProblem ==
  data: VehicleDynamicState input Bus: VehicleDynamicState; dot_d_numerical input; PathPos input; f output size=[2*(sys.N_hor+1)+sys.ns_total,1]; lb output size=[sys.n_constr*sys.N_hor+sys.n_sys+sys.m_sys+sys.ns_total,1]; ub output size=[sys.n_constr*sys.N_hor+sys.n_sys+sys.m_sys+sys.ns_total,1]; A_x output size=[1 sys.A_nnz]; v_traj input; ax_diff_traj input; ax_traj input size=sys.N_hor+1; ay_traj input size=sys.N_hor+1; ax_lim_mps2 input; ay_lim_mps2 input; tube_r_m input; tube_l_m input; d_Target_m input; dot_d_Target_mps input; vx_lin input; kappa_lin input; UncertaintyTube input; v_terminal_mps input; ax_traj_old input; ay_traj_old input; solution_old input; sys parameter; be_u_abs output; be_l_abs output; s_current_m output; P_VDC_VirtualController parameter; drag_coefficient parameter; roh_air parameter; vehiclemass_kg parameter; error_state output; P_VDC_PositiveAxLimScale parameter; P_VDC_EnableNumLatErrorDer_b parameter; P_VDC_MaxTightening parameter; P_VDC_MinVelSlipCalc_mps parameter
function [f, lb, ub, A_x, be_u_abs, be_l_abs, s_current_m, error_state]  = ...
    prepareOptimizationProblem(VehicleDynamicState, dot_d_numerical, PathPos, v_traj, ...
    ax_diff_traj, ax_traj, ay_traj, ax_lim_mps2, ay_lim_mps2, ...
    tube_r_m, tube_l_m, d_Target_m, dot_d_Target_mps, ...
    vx_lin, kappa_lin, UncertaintyTube, v_terminal_mps, ax_traj_old, ay_traj_old, solution_old, ...
    sys, P_VDC_VirtualController, drag_coefficient, roh_air, vehiclemass_kg, ...
    P_VDC_PositiveAxLimScale, P_VDC_EnableNumLatErrorDer_b, P_VDC_MaxTightening, ...
    P_VDC_MinVelSlipCalc_mps)

[f, lb, ub, A_x, be_u_abs, be_l_abs, s_current_m, error_state] =...
    prepareOptimizationProblem(VehicleDynamicState, dot_d_numerical, PathPos, v_traj, ...
    ax_diff_traj, ax_traj, ay_traj, ...
    ax_lim_mps2, ay_lim_mps2, tube_r_m, tube_l_m, d_Target_m, dot_d_Target_mps, ...
    vx_lin, kappa_lin, UncertaintyTube, v_terminal_mps, ax_traj_old, ay_traj_old, solution_old, ...
    sys, P_VDC_VirtualController, drag_coefficient, roh_air, vehiclemass_kg, ...
    P_VDC_PositiveAxLimScale, P_VDC_EnableNumLatErrorDer_b, P_VDC_MaxTightening, ...
    P_VDC_MinVelSlipCalc_mps);

end

== matlab function mvdc_mpc/AccelerationControllers/LateralController/Feedforward_Learning/Subsystem/MATLAB Function ==
  data: v input; y_meas input; w_upd output; w_old input; P_old input; P_upd output; acc_control_learning parameter; mean_debug output; cov_debug output
function [w_upd, P_upd, mean_debug, cov_debug] = learnRLSModel(v, y_meas, w_old, P_old, acc_control_learning)
    [w_upd, P_upd, mean_debug, cov_debug] = learnRLSModel(v, y_meas, w_old, P_old, acc_control_learning);

== matlab function mvdc_mpc/MPC/TubeMPC/prepareLinearization ==
  data: VehicleDynamicState input; flag_s_request output; PathPos output Bus: PathPos; TargetTrajectory input; M_tilde input; LatAcc_P_cov input; s_dot_pred_old input; vx_pred_old input; vx_lin_old input; s_dot_lin_old input; x_traj output; y_traj output; psi_traj output; v_traj output; kappa_traj output; ax_diff_traj output; ax_traj output; ay_traj output; ax_lim_mps2_tartraj output; ay_lim_mps2_tartraj output; tube_r_m output; tube_l_m output; d_Target_m output; dot_d_Target_mps output; d_lim_ub_m output; d_lim_lb_m output; ax_dist_mps2 output; ay_dist_mps2 output; vx_lin output; s_dot_lin output; kappa_lin output; P_VDC_MinVelSlipCalc_mps parameter; P_VDC_RTISQP_alpha_old parameter; P_VDC_RTISQP_alpha_target parameter; P_VDC_IncreaseUncertaintyPerStep_perc parameter; P_VDC_ControlMargin_ax_mps2 parameter; P_VDC_ControlMargin_ay_mps2 parameter; sys parameter; UncertaintyTube output; P_VDC_VirtualController parameter; acc_control_learning parameter; v_terminal_mps output; P_VDC_TerminalSetBrakeTime_s parameter; drag_coefficient parameter; roh_air parameter; vehiclemass_kg parameter; P_VDC_TuneTerminalSet_mps parameter
function [flag_s_request, PathPos, x_traj, y_traj, psi_traj, v_traj, kappa_traj, ...
    ax_diff_traj, ax_traj, ay_traj, ax_lim_mps2_tartraj, ay_lim_mps2_tartraj, ...
    tube_r_m, tube_l_m, d_Target_m, dot_d_Target_mps, ...
    d_lim_ub_m, d_lim_lb_m, ax_dist_mps2, ay_dist_mps2, ...
    vx_lin, s_dot_lin, kappa_lin, UncertaintyTube, v_terminal_mps] = ...
    prepareLinearization(VehicleDynamicState, TargetTrajectory, M_tilde, LatAcc_P_cov, ...
    s_dot_pred_old, vx_pred_old, vx_lin_old, s_dot_lin_old, P_VDC_MinVelSlipCalc_mps, P_VDC_RTISQP_alpha_old, P_VDC_RTISQP_alpha_target, ...
    P_VDC_IncreaseUncertaintyPerStep_perc, P_VDC_ControlMargin_ax_mps2, P_VDC_ControlMargin_ay_mps2, ...
    sys, P_VDC_VirtualController, acc_control_learning, ...
    P_VDC_TerminalSetBrakeTime_s, drag_coefficient, roh_air, vehiclemass_kg, ...
    P_VDC_TuneTerminalSet_mps)

[flag_s_request, PathPos, x_traj, y_traj, psi_traj, v_traj, kappa_traj, ...
    ax_diff_traj, ax_traj, ay_traj, ax_lim_mps2_tartraj, ay_lim_mps2_tartraj, ...
    tube_r_m, tube_l_m, d_Target_m, dot_d_Target_mps, ...
    d_lim_ub_m, d_lim_lb_m, ax_dist_mps2, ay_dist_mps2, ...
    vx_lin, s_dot_lin, kappa_lin, UncertaintyTube, v_terminal_mps] = ...
    prepareLinearization(VehicleDynamicState, TargetTrajectory, M_tilde, LatAcc_P_cov, ...
    s_dot_pred_old, vx_pred_old, s_dot_lin_old, vx_lin_old, sys, ...
    P_VDC_MinVelSlipCalc_mps, P_VDC_RTISQP_alpha_old, P_VDC_RTISQP_alpha_target, ...
    P_VDC_IncreaseUncertaintyPerStep_perc, P_VDC_VirtualController, ...
    P_VDC_ControlMargin_ax_mps2, P_VDC_ControlMargin_ay_mps2, acc_control_learning, ...
    P_VDC_TerminalSetBrakeTime_s, drag_coefficient, roh_air, vehiclemass_kg, ...
    P_VDC_TuneTerminalSet_mps);
